simulink model "CryoDetHcd2x"  (R2016b)
settings: Solver=ode45  StartTime=0.0  StopTime=10.0  RelTol=1e-3
PreLoadFcn:
  | setup_hcd_2x
values from neighbouring files (symbols this model uses):
  analysis_coefficients = [analysis_coefficients, fliplr(filts(i,:))]    [setup_hcd.m]
  axi_clk = 156.25e6    (= 156250000)    [setup_hcd.m]
  Fadc = 614e6    (= 614000000)    [setup_hcd.m]
  synthesis_coefficients = [synthesis_coefficients, filts(i,:)]    [setup_hcd.m]
undefined symbols (not defined in the file or in its folder): AXI4, j, Lite
libraries: xbsIndex_r4 x251
(part 2 of 2)

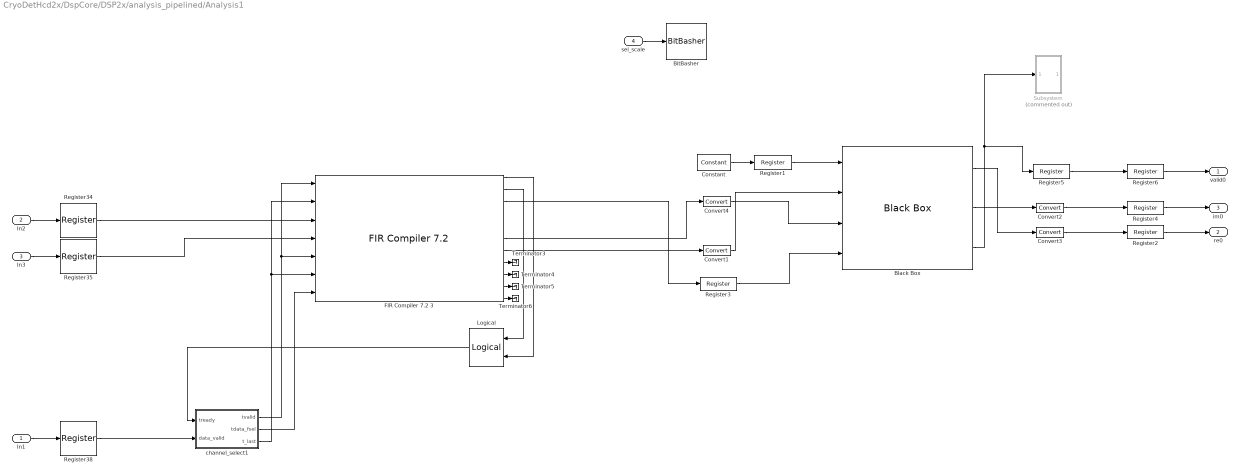
== system CryoDetHcd2x/DspCore/DSP2x/analysis_pipelined/Analysis1 ==
  In1 : Inport
  In2 : Inport  Port=2
  In3 : Inport  Port=3
  sel_scale : Inport  Port=4
  BitBasher : xbsIndex_r4/BitBasher  bitexpr=|  display_expr=off  sr_1=sel0  arith_type1=Unsigned  bin_pt1=0  sr_2=sel1  arith_type2=Unsigned  bin_pt2=0  sr_3=3  arith_type3=Unsigned  bin_pt3=0  sr_4=4  arith_type4=Unsigned  bin_pt4=0  dbl_ovrd=off  block_type=bitbasher
      | sel0 = {in[0]}
      | sel1 = {in[1]}
  Black Box : xbsIndex_r4/Black Box  init_code=IFFT_config  sim_method=ISE Simulator  verbose=off  block_type=blackbox2
  Constant : xbsIndex_r4/Constant  const=0  gui_display_data_type=Fixed-point  arith_type=Unsigned  n_bits=1  bin_pt=0  preci_type=Single  exp_width=8  frac_width=24  explicit_period=on  period=1/Fadc  equ=P=C  opselect=C  inp2=PCIN>>17  opr=+  inp1=P  carry=CIN  dbl_ovrd=off  block_type=constant
  Convert1 : xbsIndex_r4/Convert  gui_display_data_type=Fixed-point  arith_type="Signed  (2's comp)"  n_bits=16  bin_pt=15  float_type=Single  exp_bits=8  fraction_bits=24  quantization="Round  (unbiased: +/- Inf)"  overflow=Wrap  en=off  latency=1  pipeline=off  dbl_ovrd=off  block_type=convert
  Convert2 : xbsIndex_r4/Convert  gui_display_data_type=Fixed-point  arith_type="Signed  (2's comp)"  n_bits=16  bin_pt=15  float_type=Single  exp_bits=8  fraction_bits=24  quantization=Truncate  overflow=Wrap  en=off  latency=1  pipeline=off  dbl_ovrd=off  block_type=convert
  Convert3 : xbsIndex_r4/Convert  gui_display_data_type=Fixed-point  arith_type="Signed  (2's comp)"  n_bits=16  bin_pt=15  float_type=Single  exp_bits=8  fraction_bits=24  quantization=Truncate  overflow=Wrap  en=off  latency=1  pipeline=off  dbl_ovrd=off  block_type=convert
  Convert4 : xbsIndex_r4/Convert  gui_display_data_type=Fixed-point  arith_type="Signed  (2's comp)"  n_bits=16  bin_pt=15  float_type=Single  exp_bits=8  fraction_bits=24  quantization="Round  (unbiased: +/- Inf)"  overflow=Wrap  en=off  latency=1  pipeline=off  dbl_ovrd=off  block_type=convert
  FIR Compiler 7.2 3 : xbsIndex_r4/FIR Compiler 7.2   coefficientvector=analysis_coefficients(:)  coefficient_sets=16  coefficient_reload=off  filter_type=Single_Rate  rate_change_type=Integer  interpolation_rate=1  decimation_rate=1  zero_pack_factor=1  channel_sequence=Basic  number_channels=16  pattern_list='P4-0,P4-1,P4-2,P4-3,P4-4'  number_paths=2  ratespecification=Output_Sample_Period  sampleperiod=1.00000000  hardwareoversamplingrate=1  coefficient_sign=Signed  quantization=Quantize_Only  coefficient_width=25  bestprecision=on  coefficient_fractional_bits=28  coefficient_structure=Inferred  output_rounding_mode=Convergent_Rounding_to_Even  output_width=20  filter_architecture=Systolic_Multiply_Accumulate  optimization_goal=Speed  optimization_list='Data_Path_Fanout,Pre-Adder_Pipeline,Coefficient_Fanout,Control_Path_Fanout,Control_Column_Fanout,Control_Broadcast_Fanout,Control_LUT_Pipeline,No_BRAM_Read_First_Mode,Optimal_Column_Lengths,Other'  data_buffer_type=Automatic  coefficient_buffer_type=Automatic  input_buffer_type=Automatic  output_buffer_type=Automatic  preference_for_other_storage=Automatic  multi_column_support=Automatic  columnconfig='16'  inter_column_pipe_length=4  data_has_tlast=Vector_Framing  m_data_has_tready=off  s_data_has_fifo=off  s_data_has_tuser=Not_Required  m_data_has_tuser=Chan_ID_Field  s_config_sync_mode=On_Vector  s_config_method=By_Channel  num_reload_slots=1  has_aclken=off  has_aresetn=off  infoeditControl=ARESETn must be asserted for a minimum of 2 cycles  reset_data_vector=on  trim_axipin_name=on  simulation_type=hybrid_sim  simulation_model=sysgen:xfirv7_2_cmodel  data_path_portlist={ 's_axis_data_tdata', 'm_axis_data_tdata' }  passband_min=0.0  passband_max=0.5  stopband_min=0.5  stopband_max=1.0  filter_selection=1  gui_behaviour='Sysgen_GUI'  data_sign=Signed  data_width=16  data_fractional_bits=0  data_tuser_width=1  wrapper_available=true  ip_wrap_arbitrary_binary_point=true  ip_name=FIR Compiler  ip_version=7.2  dsptool_ready=true  ipcore_usecache=true  ipcore_useipmodelcache=true  port_translation_map={ 'aclken' => 'en', 'aresetn' => 'rst' }  run_core_at_system_period=true  ipcore_xco_need_fpga_part=true  block_type=fir_compiler_v7_2
      settings: infoedit=Maximum Possible : Maximizes oversampling rate. Abstracted input handshake (no s_data_tvalid) and automatic rate propagation.<br>Hardware Oversampling Rate : Specifies oversampling rate relative to the input sample period. Abstracted input handshake (no s_data_tvalid) and automatic rate propagation.<br>Input/Output Sample Period : Specifies absolute oversampling rate. No input handshake abstraction (exposes s_data_tvalid) and no rate propagation.
  Logical : xbsIndex_r4/Logical  logical_function=AND  inputs=2  en=off  latency=1  precision=Full  arith_type=Unsigned  n_bits=16  bin_pt=0  align_bp=on  dbl_ovrd=off  block_type=logical
  Register1 : xbsIndex_r4/Register  init=1  rst=off  en=off  dbl_ovrd=off  block_type=register
  Register{2..6,34..35,38} (8 alike) : xbsIndex_r4/Register  init=0  rst=off  en=off  dbl_ovrd=off  block_type=register
  Subsystem : Subsystem  Commented=on
  Terminator{3..6} (4 alike) : Terminator
  channel_select1 : Subsystem
  valid0 : Outport
  re0 : Outport  Port=2
  im0 : Outport  Port=3
  wires:
  Register5/1 -> Register6/1
  Register4/1 -> im0/1
  Register2/1 -> re0/1
  Black Box/3 -> Subsystem/1(In1), Register5/1
  Register1/1 -> Black Box/1
  Constant/1 -> Register1/1
  Register3/1 -> Black Box/4
  Convert1/1 -> Black Box/2
  Convert4/1 -> Black Box/3
  Convert3/1 -> Register2/1
  Convert2/1 -> Register4/1
  Register6/1 -> valid0/1
  Black Box/2 -> Convert2/1
  Black Box/1 -> Convert3/1
  FIR Compiler 7.2 3/3 -> Register3/1
  FIR Compiler 7.2 3/7 -> Convert1/1
  FIR Compiler 7.2 3/6 -> Convert4/1
  sel_scale/1 -> BitBasher/1
  Register38/1 -> channel_select1/2(data_valid)
  Register35/1 -> FIR Compiler 7.2 3/4
  Register34/1 -> FIR Compiler 7.2 3/3
  In2/1 -> Register34/1
  channel_select1/3(t_last) -> FIR Compiler 7.2 3/6, FIR Compiler 7.2 3/2
  FIR Compiler 7.2 3/11 -> Terminator6/1
  FIR Compiler 7.2 3/10 -> Terminator5/1
  FIR Compiler 7.2 3/9 -> Terminator4/1
  FIR Compiler 7.2 3/8 -> Terminator3/1
  FIR Compiler 7.2 3/2 -> Logical/1
  FIR Compiler 7.2 3/1 -> Logical/2
  Logical/1 -> channel_select1/1(tready)
  In1/1 -> Register38/1
  In3/1 -> Register35/1
  channel_select1/1(tvalid) -> FIR Compiler 7.2 3/1, FIR Compiler 7.2 3/5
  channel_select1/2(tdata_fsel) -> FIR Compiler 7.2 3/7

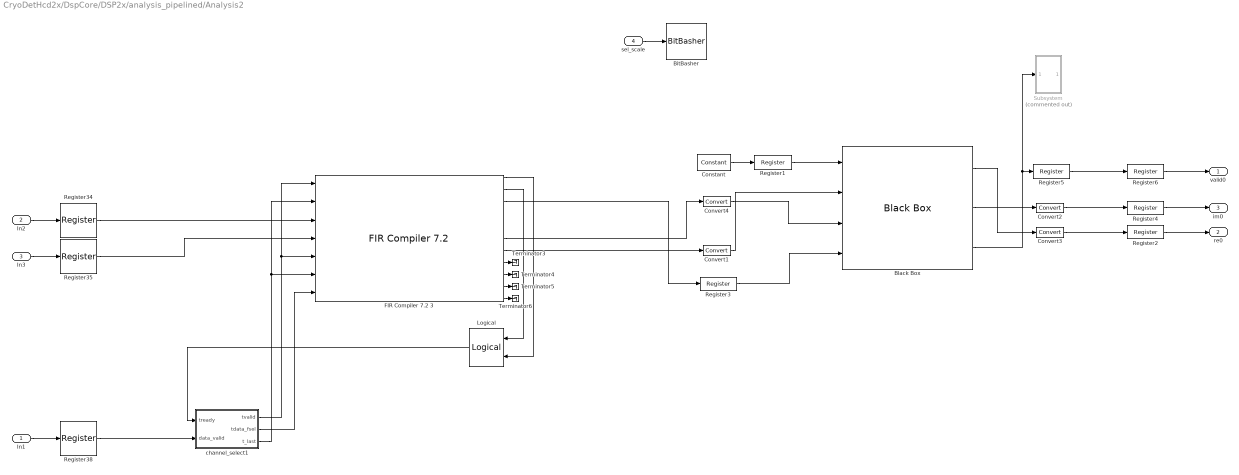
== system CryoDetHcd2x/DspCore/DSP2x/analysis_pipelined/Analysis2 ==
  In1 : Inport
  In2 : Inport  Port=2
  In3 : Inport  Port=3
  sel_scale : Inport  Port=4
  BitBasher : xbsIndex_r4/BitBasher  bitexpr=|  display_expr=off  sr_1=sel0  arith_type1=Unsigned  bin_pt1=0  sr_2=sel1  arith_type2=Unsigned  bin_pt2=0  sr_3=3  arith_type3=Unsigned  bin_pt3=0  sr_4=4  arith_type4=Unsigned  bin_pt4=0  dbl_ovrd=off  block_type=bitbasher
      | sel0 = {in[0]}
      | sel1 = {in[1]}
  Black Box : xbsIndex_r4/Black Box  init_code=IFFT_config  sim_method=ISE Simulator  verbose=off  block_type=blackbox2
  Constant : xbsIndex_r4/Constant  const=0  gui_display_data_type=Fixed-point  arith_type=Unsigned  n_bits=1  bin_pt=0  preci_type=Single  exp_width=8  frac_width=24  explicit_period=on  period=1/Fadc  equ=P=C  opselect=C  inp2=PCIN>>17  opr=+  inp1=P  carry=CIN  dbl_ovrd=off  block_type=constant
  Convert1 : xbsIndex_r4/Convert  gui_display_data_type=Fixed-point  arith_type="Signed  (2's comp)"  n_bits=16  bin_pt=15  float_type=Single  exp_bits=8  fraction_bits=24  quantization="Round  (unbiased: +/- Inf)"  overflow=Wrap  en=off  latency=1  pipeline=off  dbl_ovrd=off  block_type=convert
  Convert2 : xbsIndex_r4/Convert  gui_display_data_type=Fixed-point  arith_type="Signed  (2's comp)"  n_bits=16  bin_pt=15  float_type=Single  exp_bits=8  fraction_bits=24  quantization=Truncate  overflow=Wrap  en=off  latency=1  pipeline=off  dbl_ovrd=off  block_type=convert
  Convert3 : xbsIndex_r4/Convert  gui_display_data_type=Fixed-point  arith_type="Signed  (2's comp)"  n_bits=16  bin_pt=15  float_type=Single  exp_bits=8  fraction_bits=24  quantization=Truncate  overflow=Wrap  en=off  latency=1  pipeline=off  dbl_ovrd=off  block_type=convert
  Convert4 : xbsIndex_r4/Convert  gui_display_data_type=Fixed-point  arith_type="Signed  (2's comp)"  n_bits=16  bin_pt=15  float_type=Single  exp_bits=8  fraction_bits=24  quantization="Round  (unbiased: +/- Inf)"  overflow=Wrap  en=off  latency=1  pipeline=off  dbl_ovrd=off  block_type=convert
  FIR Compiler 7.2 3 : xbsIndex_r4/FIR Compiler 7.2   coefficientvector=analysis_coefficients(:)  coefficient_sets=16  coefficient_reload=off  filter_type=Single_Rate  rate_change_type=Integer  interpolation_rate=1  decimation_rate=1  zero_pack_factor=1  channel_sequence=Basic  number_channels=16  pattern_list='P4-0,P4-1,P4-2,P4-3,P4-4'  number_paths=2  ratespecification=Output_Sample_Period  sampleperiod=1.00000000  hardwareoversamplingrate=1  coefficient_sign=Signed  quantization=Quantize_Only  coefficient_width=25  bestprecision=on  coefficient_fractional_bits=28  coefficient_structure=Inferred  output_rounding_mode=Convergent_Rounding_to_Even  output_width=20  filter_architecture=Systolic_Multiply_Accumulate  optimization_goal=Speed  optimization_list='Data_Path_Fanout,Pre-Adder_Pipeline,Coefficient_Fanout,Control_Path_Fanout,Control_Column_Fanout,Control_Broadcast_Fanout,Control_LUT_Pipeline,No_BRAM_Read_First_Mode,Optimal_Column_Lengths,Other'  data_buffer_type=Automatic  coefficient_buffer_type=Automatic  input_buffer_type=Automatic  output_buffer_type=Automatic  preference_for_other_storage=Automatic  multi_column_support=Automatic  columnconfig='16'  inter_column_pipe_length=4  data_has_tlast=Vector_Framing  m_data_has_tready=off  s_data_has_fifo=off  s_data_has_tuser=Not_Required  m_data_has_tuser=Chan_ID_Field  s_config_sync_mode=On_Vector  s_config_method=By_Channel  num_reload_slots=1  has_aclken=off  has_aresetn=off  infoeditControl=ARESETn must be asserted for a minimum of 2 cycles  reset_data_vector=on  trim_axipin_name=on  simulation_type=hybrid_sim  simulation_model=sysgen:xfirv7_2_cmodel  data_path_portlist={ 's_axis_data_tdata', 'm_axis_data_tdata' }  passband_min=0.0  passband_max=0.5  stopband_min=0.5  stopband_max=1.0  filter_selection=1  gui_behaviour='Sysgen_GUI'  data_sign=Signed  data_width=16  data_fractional_bits=0  data_tuser_width=1  wrapper_available=true  ip_wrap_arbitrary_binary_point=true  ip_name=FIR Compiler  ip_version=7.2  dsptool_ready=true  ipcore_usecache=true  ipcore_useipmodelcache=true  port_translation_map={ 'aclken' => 'en', 'aresetn' => 'rst' }  run_core_at_system_period=true  ipcore_xco_need_fpga_part=true  block_type=fir_compiler_v7_2
      settings: infoedit=Maximum Possible : Maximizes oversampling rate. Abstracted input handshake (no s_data_tvalid) and automatic rate propagation.<br>Hardware Oversampling Rate : Specifies oversampling rate relative to the input sample period. Abstracted input handshake (no s_data_tvalid) and automatic rate propagation.<br>Input/Output Sample Period : Specifies absolute oversampling rate. No input handshake abstraction (exposes s_data_tvalid) and no rate propagation.
  Logical : xbsIndex_r4/Logical  logical_function=AND  inputs=2  en=off  latency=1  precision=Full  arith_type=Unsigned  n_bits=16  bin_pt=0  align_bp=on  dbl_ovrd=off  block_type=logical
  Register1 : xbsIndex_r4/Register  init=1  rst=off  en=off  dbl_ovrd=off  block_type=register
  Register{2..6,34..35,38} (8 alike) : xbsIndex_r4/Register  init=0  rst=off  en=off  dbl_ovrd=off  block_type=register
  Subsystem : Subsystem  Commented=on
  Terminator{3..6} (4 alike) : Terminator
  channel_select1 : Subsystem
  valid0 : Outport
  re0 : Outport  Port=2
  im0 : Outport  Port=3
  wires:
  channel_select1/2(tdata_fsel) -> FIR Compiler 7.2 3/7
  channel_select1/1(tvalid) -> FIR Compiler 7.2 3/5, FIR Compiler 7.2 3/1
  In3/1 -> Register35/1
  In1/1 -> Register38/1
  Logical/1 -> channel_select1/1(tready)
  FIR Compiler 7.2 3/1 -> Logical/2
  FIR Compiler 7.2 3/2 -> Logical/1
  FIR Compiler 7.2 3/8 -> Terminator3/1
  FIR Compiler 7.2 3/9 -> Terminator4/1
  FIR Compiler 7.2 3/10 -> Terminator5/1
  FIR Compiler 7.2 3/11 -> Terminator6/1
  channel_select1/3(t_last) -> FIR Compiler 7.2 3/2, FIR Compiler 7.2 3/6
  In2/1 -> Register34/1
  Register34/1 -> FIR Compiler 7.2 3/3
  Register35/1 -> FIR Compiler 7.2 3/4
  Register38/1 -> channel_select1/2(data_valid)
  sel_scale/1 -> BitBasher/1
  FIR Compiler 7.2 3/6 -> Convert4/1
  FIR Compiler 7.2 3/7 -> Convert1/1
  FIR Compiler 7.2 3/3 -> Register3/1
  Black Box/1 -> Convert3/1
  Black Box/2 -> Convert2/1
  Register6/1 -> valid0/1
  Convert2/1 -> Register4/1
  Convert3/1 -> Register2/1
  Convert4/1 -> Black Box/3
  Convert1/1 -> Black Box/2
  Register3/1 -> Black Box/4
  Constant/1 -> Register1/1
  Register1/1 -> Black Box/1
  Black Box/3 -> Subsystem/1(In1), Register5/1
  Register2/1 -> re0/1
  Register4/1 -> im0/1
  Register5/1 -> Register6/1

== system CryoDetHcd2x/DspCore/DSP2x/analysis_pipelined/Pre-Analysis0 ==
  valid : Inport
  im : Inport  Port=2
  re : Inport  Port=3
  Delay : xbsIndex_r4/Delay  rst=off  infoeditControl=Selection of Reset will increase slice count due to use of real FFs and instead of SRLs  en=off  latency=9  reg_retiming=off  dbl_ovrd=off  block_type=delay
  Delay1 : xbsIndex_r4/Delay  rst=off  infoeditControl=Selection of Reset will increase slice count due to use of real FFs and instead of SRLs  en=off  latency=9  reg_retiming=off  dbl_ovrd=off  block_type=delay
  Delay2 : xbsIndex_r4/Delay  rst=off  infoeditControl=Selection of Reset will increase slice count due to use of real FFs and instead of SRLs  en=off  latency=9  reg_retiming=off  dbl_ovrd=off  block_type=delay
  valid0 : Outport
  im0 : Outport  Port=2
  reo : Outport  Port=3
  wires:
  Delay2/1 -> reo/1
  Delay1/1 -> im0/1
  Delay/1 -> valid0/1
  re/1 -> Delay2/1
  im/1 -> Delay1/1
  valid/1 -> Delay/1

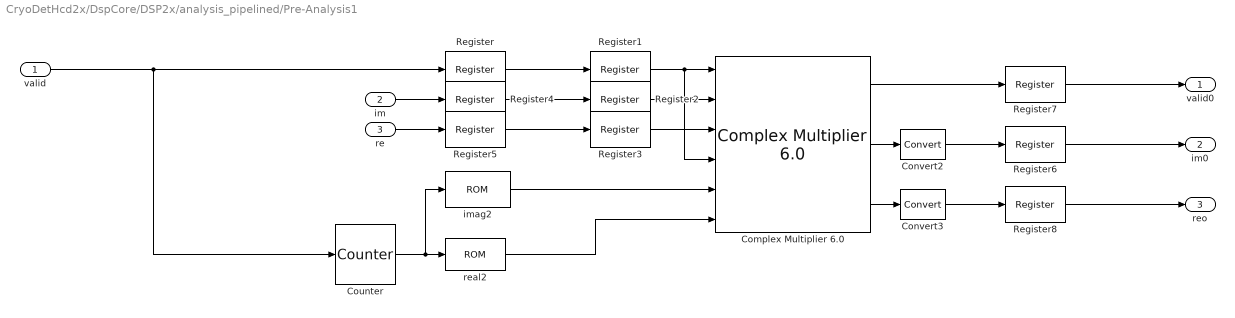
== system CryoDetHcd2x/DspCore/DSP2x/analysis_pipelined/Pre-Analysis1 ==
  valid : Inport
  im : Inport  Port=2
  re : Inport  Port=3
  "Complex Multiplier 6.0 " : xbsIndex_r4/Complex Multiplier 6.0   hasatlast=off  hasatuser=off  atuserwidth=1  hasbtlast=off  hasbtuser=off  btuserwidth=1  multtype=Use_Mults  optimizegoal=Performance  flowcontrol=NonBlocking  outputwidth=19  roundmode=Truncate  hasctrltlast=off  hasctrltuser=off  ctrltuserwidth=1  outtlastbehv=Null  latencyconfig=Automatic  minimumlatency=34  aclken=off  aresetn=off  trim_axipin_name=on  simulation_type=hybrid_sim  simulation_model=sysgen:cmpy_v6_0  data_path_portlist={ 's_axis_a_tdata_real', 's_axis_a_tdata_imag', 's_axis_b_tdata_real', 's_axis_b_tdata_imag', 's_axis_ctrl_tdata_rounding_bit', 'm_axis_dout_tdata_real', 'm_axis_dout_tdata_imag' }  aportwidth=63  bportwidth=63  ip_name=Complex Multiplier  ip_version=6.0  dsptool_ready=true  ipcore_usecache=true  ipcore_useipmodelcache=true  ipcore_verbose=false  ipcore_latency_parameter='minimumlatency'  wrapper_available=true  port_translation_map={ 'aclken' => 'en', 'aresetn' => 'rst'}  block_type=cmpy_v6_0
  Convert2 : xbsIndex_r4/Convert  gui_display_data_type=Fixed-point  arith_type="Signed  (2's comp)"  n_bits=16  bin_pt=15  float_type=Single  exp_bits=8  fraction_bits=24  quantization=Truncate  overflow=Flag as error  en=off  latency=0  pipeline=off  dbl_ovrd=off  block_type=convert
  Convert3 : xbsIndex_r4/Convert  gui_display_data_type=Fixed-point  arith_type="Signed  (2's comp)"  n_bits=16  bin_pt=15  float_type=Single  exp_bits=8  fraction_bits=24  quantization=Truncate  overflow=Flag as error  en=off  latency=0  pipeline=off  dbl_ovrd=off  block_type=convert
  Counter : xbsIndex_r4/Counter  cnt_type=Free Running  cnt_to=Inf  operation=Up  start_count=0  cnt_by_val=1  arith_type=Unsigned  n_bits=5  bin_pt=0  load_pin=off  rst=off  en=on  explicit_period=on  period=1/Fadc  use_behavioral_HDL=off  implementation=Fabric  dbl_ovrd=off  block_type=counter
  Register{,1..8} (9 alike) : xbsIndex_r4/Register  init=0  rst=off  en=off  dbl_ovrd=off  block_type=register
  imag2 : xbsIndex_r4/ROM  depth=32  initVector=imag(exp(-j*2*pi*(0:1:31)/32))  distributed_mem=Block RAM  rst=off  init_reg=0  en=off  latency=2  gui_display_data_type=Fixed-point  arith_type="Signed  (2's comp)"  n_bits=18  bin_pt=16  preci_type=Single  exp_width=8  frac_width=24  optimize=Area  use_rpm=on  dbl_ovrd=off  block_type=sprom
  real2 : xbsIndex_r4/ROM  depth=32  initVector=real(exp(-j*2*pi*(0:1:31)/32))  distributed_mem=Block RAM  rst=off  init_reg=0  en=off  latency=2  gui_display_data_type=Fixed-point  arith_type="Signed  (2's comp)"  n_bits=18  bin_pt=16  preci_type=Single  exp_width=8  frac_width=24  optimize=Area  use_rpm=on  dbl_ovrd=off  block_type=sprom
  valid0 : Outport
  im0 : Outport  Port=2
  reo : Outport  Port=3
  wires:
  real2/1 -> "Complex Multiplier 6.0 "/6
  imag2/1 -> "Complex Multiplier 6.0 "/5
  Register3/1 -> "Complex Multiplier 6.0 "/3
  Register2/1 -> "Complex Multiplier 6.0 "/2
  Register1/1 -> "Complex Multiplier 6.0 "/1, "Complex Multiplier 6.0 "/4
  "Complex Multiplier 6.0 "/1 -> Register7/1
  Register/1 -> Register1/1
  valid/1 -> Counter/1, Register/1
  Counter/1 -> real2/1, imag2/1
  re/1 -> Register5/1
  Register4/1 -> Register2/1
  Register5/1 -> Register3/1
  "Complex Multiplier 6.0 "/3 -> Convert3/1
  "Complex Multiplier 6.0 "/2 -> Convert2/1
  Convert2/1 -> Register6/1
  Convert3/1 -> Register8/1
  im/1 -> Register4/1
  Register6/1 -> im0/1
  Register7/1 -> valid0/1
  Register8/1 -> reo/1

== system CryoDetHcd2x/DspCore/DSP2x/Synthesis/Syntehsis1/Subsystem ==
  In1 : Inport
  Adc0 : xbsIndex_r4/Gateway In  gui_display_data_type=Boolean  arith_type=Boolean  n_bits=16  bin_pt=15  preci_type=Single  exp_width=8  frac_width=24  rows=1  columns=1  quantization=Truncate  overflow=Wrap  period=1/Fadc  UseAsADC=off  ADCChannel='1'  interface=None  automatic_assignment=on  address_offset=hex2dec('00')  intf_name=''  intf_description=''  default_value=0  timing_constraint=None  locs_specified=off  LOCs={}  io_standard={}  inherit_from_input=off  hdl_port=on  dbl_ovrd=off  block_type=gatewayin
  Constant1 : xbsIndex_r4/Constant  const=0  gui_display_data_type=Boolean  arith_type=Boolean  n_bits=1  bin_pt=0  preci_type=Single  exp_width=8  frac_width=24  explicit_period=on  period=1/Fadc  equ=P=C  opselect=C  inp2=PCIN>>17  opr=+  inp1=P  carry=CIN  dbl_ovrd=off  block_type=constant
  Indeterminate Probe1 : xbsIndex_r4/Indeterminate Probe  block_type=indetprobe
      settings: infoedit=Produces an output 1 of type double when input data is indeterminate. Output is 0 otherwise.<br><br>Hardware notes: This block and any downstream blocks will be trimmed when hardware is generated.
  Mux : xbsIndex_r4/Mux  inputs=2  en=off  latency=1  precision=Full  arith_type=Unsigned  n_bits=16  bin_pt=14  quantization=Truncate  overflow=Wrap  dbl_ovrd=off  block_type=mux
  Out1 : Outport
  wires:
  In1/1 -> Indeterminate Probe1/1, Mux/2
  Constant1/1 -> Mux/3
  Adc0/1 -> Mux/1
  Mux/1 -> Out1/1
  Indeterminate Probe1/1 -> Adc0/1

== system CryoDetHcd2x/DspCore/DSP2x/Synthesis/Syntehsis2/Subsystem ==
  In1 : Inport
  Adc0 : xbsIndex_r4/Gateway In  gui_display_data_type=Boolean  arith_type=Boolean  n_bits=16  bin_pt=15  preci_type=Single  exp_width=8  frac_width=24  rows=1  columns=1  quantization=Truncate  overflow=Wrap  period=1/Fadc  UseAsADC=off  ADCChannel='1'  interface=None  automatic_assignment=on  address_offset=hex2dec('00')  intf_name=''  intf_description=''  default_value=0  timing_constraint=None  locs_specified=off  LOCs={}  io_standard={}  inherit_from_input=off  hdl_port=on  dbl_ovrd=off  block_type=gatewayin
  Constant1 : xbsIndex_r4/Constant  const=0  gui_display_data_type=Boolean  arith_type=Boolean  n_bits=1  bin_pt=0  preci_type=Single  exp_width=8  frac_width=24  explicit_period=on  period=1/Fadc  equ=P=C  opselect=C  inp2=PCIN>>17  opr=+  inp1=P  carry=CIN  dbl_ovrd=off  block_type=constant
  Indeterminate Probe1 : xbsIndex_r4/Indeterminate Probe  block_type=indetprobe
      settings: infoedit=Produces an output 1 of type double when input data is indeterminate. Output is 0 otherwise.<br><br>Hardware notes: This block and any downstream blocks will be trimmed when hardware is generated.
  Mux : xbsIndex_r4/Mux  inputs=2  en=off  latency=1  precision=Full  arith_type=Unsigned  n_bits=16  bin_pt=14  quantization=Truncate  overflow=Wrap  dbl_ovrd=off  block_type=mux
  Out1 : Outport
  wires:
  Indeterminate Probe1/1 -> Adc0/1
  Mux/1 -> Out1/1
  Adc0/1 -> Mux/1
  Constant1/1 -> Mux/3
  In1/1 -> Mux/2, Indeterminate Probe1/1

== system CryoDetHcd2x/DspCore/DSP2x/analysis_pipelined/Analysis1/Subsystem ==
  In1 : Inport
  Adc0 : xbsIndex_r4/Gateway In  gui_display_data_type=Boolean  arith_type=Boolean  n_bits=16  bin_pt=15  preci_type=Single  exp_width=8  frac_width=24  rows=1  columns=1  quantization=Truncate  overflow=Wrap  period=1/Fadc  UseAsADC=off  ADCChannel='1'  interface=None  automatic_assignment=on  address_offset=hex2dec('00')  intf_name=''  intf_description=''  default_value=0  timing_constraint=None  locs_specified=off  LOCs={}  io_standard={}  inherit_from_input=off  hdl_port=on  dbl_ovrd=off  block_type=gatewayin
  Constant1 : xbsIndex_r4/Constant  const=0  gui_display_data_type=Boolean  arith_type=Boolean  n_bits=1  bin_pt=0  preci_type=Single  exp_width=8  frac_width=24  explicit_period=on  period=1/Fadc  equ=P=C  opselect=C  inp2=PCIN>>17  opr=+  inp1=P  carry=CIN  dbl_ovrd=off  block_type=constant
  Indeterminate Probe : xbsIndex_r4/Indeterminate Probe  block_type=indetprobe
      settings: infoedit=Produces an output 1 of type double when input data is indeterminate. Output is 0 otherwise.<br><br>Hardware notes: This block and any downstream blocks will be trimmed when hardware is generated.
  Mux : xbsIndex_r4/Mux  inputs=2  en=off  latency=1  precision=Full  arith_type=Unsigned  n_bits=16  bin_pt=14  quantization=Truncate  overflow=Wrap  dbl_ovrd=off  block_type=mux
  Time Scope : Scope
  Out1 : Outport
  wires:
  Constant1/1 -> Mux/3
  Mux/1 -> Out1/1
  Indeterminate Probe/1 -> Adc0/1, Time Scope/1
  Adc0/1 -> Mux/1
  In1/1 -> Indeterminate Probe/1, Mux/2

== system CryoDetHcd2x/DspCore/DSP2x/analysis_pipelined/Analysis1/channel_select1 ==
  tready : Inport
  data_valid : Inport  Port=2
  Constant : xbsIndex_r4/Constant  const=6  gui_display_data_type=Fixed-point  arith_type=Unsigned  n_bits=3  bin_pt=0  preci_type=Single  exp_width=8  frac_width=24  explicit_period=off  period=1  equ=P=C  opselect=C  inp2=PCIN>>17  opr=+  inp1=P  carry=CIN  dbl_ovrd=off  block_type=constant
  Counter : xbsIndex_r4/Counter  cnt_type=Free Running  cnt_to=Inf  operation=Up  start_count=0  cnt_by_val=1  arith_type=Unsigned  n_bits=4  bin_pt=0  load_pin=off  rst=off  en=on  explicit_period=on  period=1/Fadc  use_behavioral_HDL=off  implementation=Fabric  dbl_ovrd=off  block_type=counter
  Logical6 : xbsIndex_r4/Logical  logical_function=AND  inputs=2  en=off  latency=1  precision=Full  arith_type=Unsigned  n_bits=16  bin_pt=0  align_bp=on  dbl_ovrd=off  block_type=logical
  Relational : xbsIndex_r4/Relational  mode=a=b  op_type=Bool  en=off  latency=1  dbl_ovrd=off  block_type=relational
  tvalid : Outport
  tdata_fsel : Outport  Port=2
  t_last : Outport  Port=3
  wires:
  Constant/1 -> Relational/1
  Relational/1 -> t_last/1
  tready/1 -> Logical6/1
  Counter/1 -> tdata_fsel/1, Relational/2
  data_valid/1 -> Logical6/2
  Logical6/1 -> Counter/1, tvalid/1

== system CryoDetHcd2x/DspCore/DSP2x/analysis_pipelined/Analysis2/Subsystem ==
  In1 : Inport
  Adc0 : xbsIndex_r4/Gateway In  gui_display_data_type=Boolean  arith_type=Boolean  n_bits=16  bin_pt=15  preci_type=Single  exp_width=8  frac_width=24  rows=1  columns=1  quantization=Truncate  overflow=Wrap  period=1/Fadc  UseAsADC=off  ADCChannel='1'  interface=None  automatic_assignment=on  address_offset=hex2dec('00')  intf_name=''  intf_description=''  default_value=0  timing_constraint=None  locs_specified=off  LOCs={}  io_standard={}  inherit_from_input=off  hdl_port=on  dbl_ovrd=off  block_type=gatewayin
  Constant1 : xbsIndex_r4/Constant  const=0  gui_display_data_type=Boolean  arith_type=Boolean  n_bits=1  bin_pt=0  preci_type=Single  exp_width=8  frac_width=24  explicit_period=on  period=1/Fadc  equ=P=C  opselect=C  inp2=PCIN>>17  opr=+  inp1=P  carry=CIN  dbl_ovrd=off  block_type=constant
  Indeterminate Probe : xbsIndex_r4/Indeterminate Probe  block_type=indetprobe
      settings: infoedit=Produces an output 1 of type double when input data is indeterminate. Output is 0 otherwise.<br><br>Hardware notes: This block and any downstream blocks will be trimmed when hardware is generated.
  Mux : xbsIndex_r4/Mux  inputs=2  en=off  latency=1  precision=Full  arith_type=Unsigned  n_bits=16  bin_pt=14  quantization=Truncate  overflow=Wrap  dbl_ovrd=off  block_type=mux
  Time Scope : Scope
  Out1 : Outport
  wires:
  In1/1 -> Mux/2, Indeterminate Probe/1
  Adc0/1 -> Mux/1
  Indeterminate Probe/1 -> Time Scope/1, Adc0/1
  Mux/1 -> Out1/1
  Constant1/1 -> Mux/3

== system CryoDetHcd2x/DspCore/DSP2x/analysis_pipelined/Analysis2/channel_select1 ==
  tready : Inport
  data_valid : Inport  Port=2
  Constant : xbsIndex_r4/Constant  const=6  gui_display_data_type=Fixed-point  arith_type=Unsigned  n_bits=3  bin_pt=0  preci_type=Single  exp_width=8  frac_width=24  explicit_period=off  period=1  equ=P=C  opselect=C  inp2=PCIN>>17  opr=+  inp1=P  carry=CIN  dbl_ovrd=off  block_type=constant
  Counter : xbsIndex_r4/Counter  cnt_type=Free Running  cnt_to=Inf  operation=Up  start_count=0  cnt_by_val=1  arith_type=Unsigned  n_bits=4  bin_pt=0  load_pin=off  rst=off  en=on  explicit_period=on  period=1/Fadc  use_behavioral_HDL=off  implementation=Fabric  dbl_ovrd=off  block_type=counter
  Logical6 : xbsIndex_r4/Logical  logical_function=AND  inputs=2  en=off  latency=1  precision=Full  arith_type=Unsigned  n_bits=16  bin_pt=0  align_bp=on  dbl_ovrd=off  block_type=logical
  Relational : xbsIndex_r4/Relational  mode=a=b  op_type=Bool  en=off  latency=1  dbl_ovrd=off  block_type=relational
  tvalid : Outport
  tdata_fsel : Outport  Port=2
  t_last : Outport  Port=3
  wires:
  Logical6/1 -> tvalid/1, Counter/1
  data_valid/1 -> Logical6/2
  Counter/1 -> Relational/2, tdata_fsel/1
  tready/1 -> Logical6/1
  Relational/1 -> t_last/1
  Constant/1 -> Relational/1
